simulink model "dyno"  (R2014a)
settings: Solver=ode45  StartTime=0.0  StopTime=6  RelTol=1e-3
libraries: embdlinuxlib x3, simulink x3
settings Model: Creator=Adam  LastModifiedBy=Adam

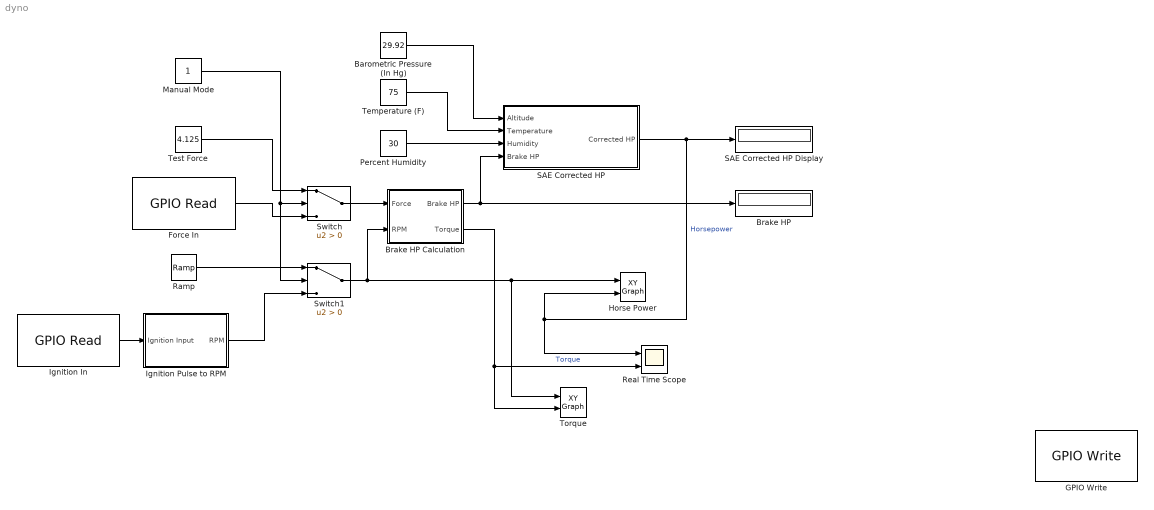
== system dyno ==
  Barometric Pressure (In Hg) : Constant  Value=29.92
  Brake HP : Display
  Brake HP Calculation : Subsystem
  Force In : embdlinuxlib/GPIO Read  board=Model B Rev2  gpio=4  internalResistor=Off  sampleTime=0.001  direction=Input  blockPlatform=Raspberry Pi
  GPIO Write : embdlinuxlib/GPIO Write  board=Model B Rev2  gpio=17  direction=Output  blockPlatform=Raspberry Pi
  Horse Power : simulink/Sinks/XY Graph  xmin=0  xmax=12500  ymin=0  ymax=200  st=-1
  Ignition In : embdlinuxlib/GPIO Read  board=Model B Rev2  gpio=9  internalResistor=Off  sampleTime=0.001  direction=Input  blockPlatform=Raspberry Pi
  Ignition Pulse to RPM : Subsystem
  Manual Mode : Constant
  Percent Humidity : Constant  Value=30
  Ramp : simulink/Sources/Ramp  slope=1700  start=0  X0=1800
  Real Time Scope : Scope  NumInputPorts=2
      settings: ShowLegends=on  TimeRange=1  YMin=52.5~25.9957  YMax=61~25.9958
  SAE Corrected HP : Subsystem
  SAE Corrected HP Display : Display
  Switch : Switch  Criteria=u2 > Threshold
  Switch1 : Switch  Criteria=u2 > Threshold
  Temperature (F) : Constant  Value=75
  Test Force : Constant  Value=4.125
  Torque : simulink/Sinks/XY Graph  xmin=0  xmax=12500  ymin=0  ymax=100  st=-1
  wires:
  Force In/1 -> Switch/3
  Switch1/1 -> Torque/1, Horse Power/1, Brake HP Calculation/2(RPM)
  Test Force/1 -> Switch/1
  Ramp/1 -> Switch1/1
  Manual Mode/1 -> Switch1/2, Switch/2
  SAE Corrected HP/1(Corrected HP) -> SAE Corrected HP Display/1, Real Time Scope/1, Horse Power/2  "Horsepower"
  Barometric Pressure (In Hg)/1 -> SAE Corrected HP/1(Altitude)
  Temperature (F)/1 -> SAE Corrected HP/2(Temperature)
  Percent Humidity/1 -> SAE Corrected HP/3(Humidity)
  Brake HP Calculation/1(Brake HP) -> Brake HP/1, SAE Corrected HP/4(Brake HP)
  Brake HP Calculation/2(Torque) -> Torque/2, Real Time Scope/2  "Torque"
  Switch/1 -> Brake HP Calculation/1(Force)
  Ignition In/1 -> Ignition Pulse to RPM/1(Ignition Input)
  Ignition Pulse to RPM/1(RPM) -> Switch1/3

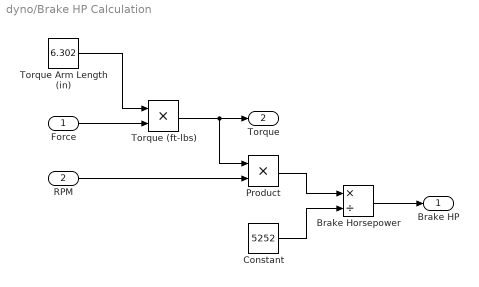
== system dyno/Brake HP Calculation ==
  Force : Inport
  RPM : Inport  Port=2
  Brake Horsepower : Product  Inputs=*/
  Constant : Constant  Value=5252
  Product : Product
  Torque (ft-lbs) : Product
  Torque Arm Length (in) : Constant  Value=6.302
  Brake HP : Outport
  Torque : Outport  Port=2
  wires:
  Constant/1 -> Brake Horsepower/2
  Brake Horsepower/1 -> Brake HP/1
  Force/1 -> Torque (ft-lbs)/2
  Product/1 -> Brake Horsepower/1
  Torque Arm Length (in)/1 -> Torque (ft-lbs)/1
  Torque (ft-lbs)/1 -> Torque/1, Product/1
  RPM/1 -> Product/2

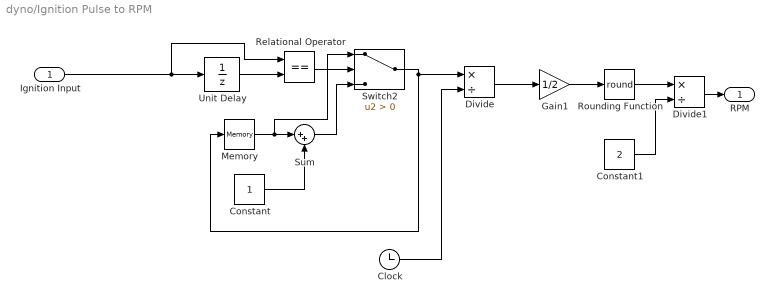
== system dyno/Ignition Pulse to RPM ==
  Ignition Input : Inport
  Clock : Clock
  Constant : Constant
  Constant1 : Constant  Value=2
  Divide : Product  Inputs=*/
  Divide1 : Product  Inputs=*/
  Gain1 : Gain  Gain=1/2
  Memory : Memory
  Relational Operator : RelationalOperator  Operator===  OutDataTypeStr=boolean
  Rounding Function : Rounding  Operator=round
  Sum : Sum  Inputs=|++
  Switch2 : Switch  Criteria=u2 > Threshold
  Unit Delay : UnitDelay  SampleTime=-1
  RPM : Outport
  wires:
  Ignition Input/1 -> Relational Operator/1, Unit Delay/1
  Memory/1 -> Sum/1, Switch2/1
  Unit Delay/1 -> Relational Operator/2
  Gain1/1 -> Rounding Function/1
  Switch2/1 -> Divide/1, Memory/1
  Constant/1 -> Sum/2
  Sum/1 -> Switch2/3
  Relational Operator/1 -> Switch2/2
  Clock/1 -> Divide/2
  Divide/1 -> Gain1/1
  Divide1/1 -> RPM/1
  Constant1/1 -> Divide1/2
  Rounding Function/1 -> Divide1/1

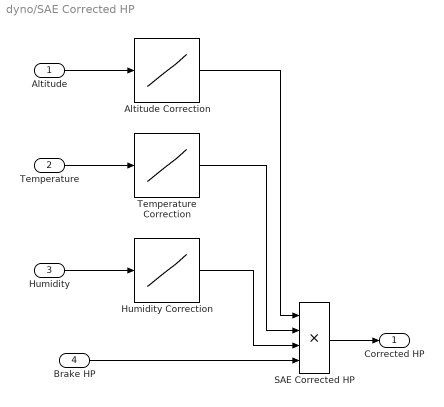
== system dyno/SAE Corrected HP ==
  Altitude : Inport
  Temperature : Inport  Port=2
  Humidity : Inport  Port=3
  Brake HP : Inport  Port=4
  Altitude Correction : Lookup_n-D  NumberOfTableDimensions=1  BreakpointsForDimension1=[19.03,19.79,20.58,21.38,22.22,23.09,23.98,24.89,25.84,26.81,27.82,28.86,29.92,30,30.1,30.20]  Table=[1.57,1.514,1.455,1.4,1.345,1.295,1.249,1.2,1.158,1.115,1.072,1.035,1,.9975,.994,0.9910]  InternalRulePriority=Speed  RndMeth=Simplest  InputSameDT=on
  Humidity Correction : Lookup_n-D  NumberOfTableDimensions=1  BreakpointsForDimension1=[10,20,30,40,50,60,70,80,90,100]  Table=[1.008,1.015,1.02,1.028,1.035,1.04,1.048,1.055,1.062,1.07]  InternalRulePriority=Speed  RndMeth=Simplest  InputSameDT=on
  SAE Corrected HP : Product  Inputs=4
  Temperature Correction : Lookup_n-D  NumberOfTableDimensions=1  BreakpointsForDimension1=[30,60,70,80,90,100,110,120,130,140,150,160,170,180,190,200]  Table=[.972,1.00,1.010,1.018,1.028,1.037,1.046,1.056,1.065,1.074,1.083,1.092,1.101,1.110,1.118,1.126]  InternalRulePriority=Speed  RndMeth=Simplest  InputSameDT=on
  Corrected HP : Outport
  wires:
  Humidity Correction/1 -> SAE Corrected HP/3
  Temperature Correction/1 -> SAE Corrected HP/2
  Altitude Correction/1 -> SAE Corrected HP/1
  SAE Corrected HP/1 -> Corrected HP/1
  Humidity/1 -> Humidity Correction/1
  Brake HP/1 -> SAE Corrected HP/4
  Altitude/1 -> Altitude Correction/1
  Temperature/1 -> Temperature Correction/1
